simulink model "model"  (R2017b)
settings: Solver=ode23tb  StartTime=0.0  StopTime=0.3  EnableMultiTasking=on
InitFcn:
  | initializer_assignment4
values from neighbouring files (symbols this model uses):
  C = 15e-06    (= 1.5e-05)    [main.m]
  Iqref = 0    [main.m]
  K_cross = (L_inv) * 2*pi*f_sin    (= 0.785398163397)    [main.m]
  Kc = 1/(w_z/K * Gc)    [main.m]
  Ki = 2776    [main.m]
  Kp = 1.165    [main.m]
  L_a_grid = L_grid    (= 0.0015)    [main.m]
  L_a_inv = L_inv    (= 0.0025)    [main.m]
  L_b_grid = L_grid    (= 0.0015)    [main.m]
  L_b_inv = L_inv    (= 0.0025)    [main.m]
  L_c_grid = L_grid    (= 0.0015)    [main.m]
  L_c_inv = L_inv    (= 0.0025)    [main.m]
  m_a = 1/Gpwm    (= 0.00285714285714)    [main.m]
  R_d = 3.1    [main.m]
  V_ac = 400    [main.m]
  w_p = w_cr * K    [main.m]
  w_ref = f_sin*2*pi    (= 314.159265359)    [main.m]
  w_z = w_cr / K    [main.m]
libraries: powerlib x20, powerlib_meascontrol x5
settings Model: Creator=Daniele  LastModifiedBy=izzy
settings SolverCC: ZeroCrossAlgorithm=Adaptive
settings DataIOCC: LimitDataPoints=on  SaveFormat=Array
settings OptimizationCC: LifeSpan=inf
settings DebuggingCC: UnderspecifiedInitializationDetection=Classic  MergeDetectMultiDrivingBlocksExec=none  SolverPrmCheckMsg=warning  SFUnexpectedBacktrackingDiag=warning  SFNoUnconditionalDefaultTransitionDiag=warning  SFExecutionAtInitializationDiag=none
settings HardwareCC: ProdBitPerPointer=32  ProdBitPerSizeT=32  ProdBitPerPtrDiffT=32  ProdLargestAtomicFloat=None  ProdIntDivRoundTo=Undefined  ProdEndianess=Unspecified  ProdWordSize=32  ProdHWDeviceType=32-bit Generic
settings ModelReferenceCC: PropagateSignalLabelsOutOfModel=off
settings CodeAppCC: StateflowObjectComments=on
settings GRTTargetCC: TargetLangStandard=C89/C90 (ANSI)  GeneratePreprocessorConditionals=Disable all
settings ConfigComp: CovMetricSettings=dw  CovHtmlReporting=on  CovSaveCumulativeToWorkspaceVar=on  CovSaveSingleToWorkspaceVar=on  CovExternalEMLEnable=off
settings SimscapeCC: SimscapeNormalizeSystem=off

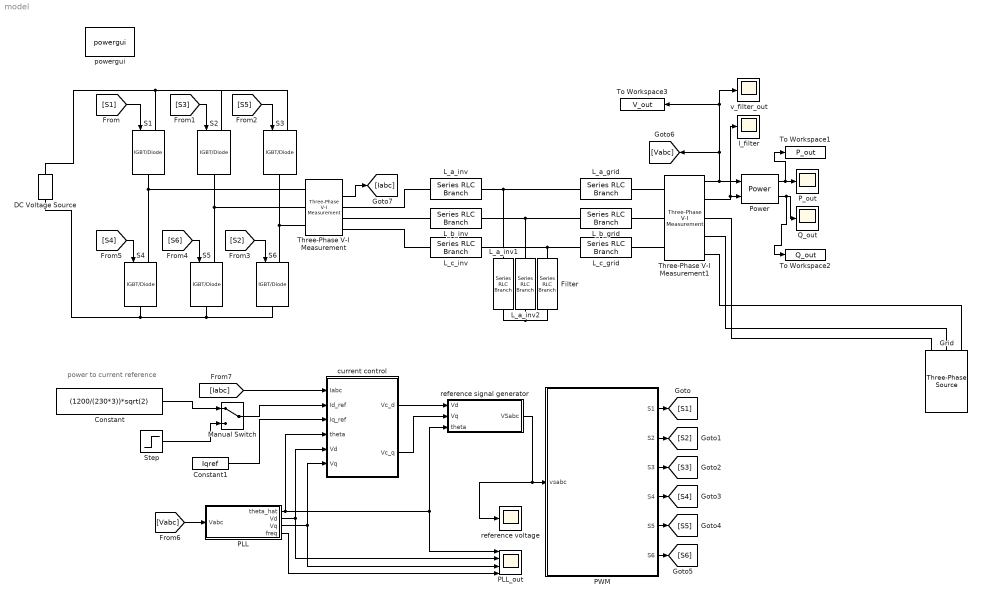
== system model ==
  note: power to current reference
  Constant : Constant  Value=(1200/(230*3))*sqrt(2)
  Constant1 : Constant  Value=Iqref
  DC Voltage Source : powerlib/Electrical Sources/DC Voltage Source  Amplitude=700  Measurements=None
  Filter : powerlib/Elements/Series RLC Branch  LConnTagsString=__new0  RConnTagsString=__new0  BranchType=RC  Resistance=R_d  Inductance=L_a_inv  SetiL0=off  InitialCurrent=0  Capacitance=C  Setx0=off  InitialVoltage=0  Measurements=None
  Grid : powerlib/Electrical Sources/Three-Phase Source  InternalConnection=Yg  VoltagePhases=off  Voltage=V_ac  PhaseAngle=0  Voltage_phases=[25e3 25e3 25e3]/sqrt(3)  PhaseAngles_phases=[0 -120 +120]  Frequency=50  NonIdealSource=on  SpecifyImpedance=off  Resistance=0.48  Inductance=250e-6  ShortCircuitLevel=100e6  BaseVoltage=V_ac  XRratio=7  BusType=swing  Pref=0  Qref=0  Prefabc=[10e3, 10e3, 10e3]  Qrefabc=[0, 0, 0]  Qmin=-inf  Qmax=inf
  I_filter : Scope
  L_a_grid : powerlib/Elements/Series RLC Branch  LConnTagsString=__new0  RConnTagsString=__new0  BranchType=L  Resistance=1  Inductance=L_a_grid  SetiL0=off  InitialCurrent=0  Capacitance=0  Setx0=off  InitialVoltage=0  Measurements=None
  L_a_inv : powerlib/Elements/Series RLC Branch  LConnTagsString=__new0  RConnTagsString=__new0  BranchType=L  Resistance=1  Inductance=L_a_inv  SetiL0=off  InitialCurrent=0  Capacitance=0  Setx0=off  InitialVoltage=0  Measurements=None
  L_a_inv1 : powerlib/Elements/Series RLC Branch  LConnTagsString=__new0  RConnTagsString=__new0  BranchType=RC  Resistance=R_d  Inductance=L_a_inv  SetiL0=off  InitialCurrent=0  Capacitance=C  Setx0=off  InitialVoltage=0  Measurements=None
  L_a_inv2 : powerlib/Elements/Series RLC Branch  LConnTagsString=__new0  RConnTagsString=__new0  BranchType=RC  Resistance=R_d  Inductance=L_a_inv  SetiL0=off  InitialCurrent=0  Capacitance=C  Setx0=off  InitialVoltage=0  Measurements=None
  L_b_grid : powerlib/Elements/Series RLC Branch  LConnTagsString=__new0  RConnTagsString=__new0  BranchType=L  Resistance=1  Inductance=L_b_grid  SetiL0=off  InitialCurrent=0  Capacitance=0  Setx0=off  InitialVoltage=0  Measurements=None
  L_b_inv : powerlib/Elements/Series RLC Branch  LConnTagsString=__new0  RConnTagsString=__new0  BranchType=L  Resistance=1  Inductance=L_b_inv  SetiL0=off  InitialCurrent=0  Capacitance=0  Setx0=off  InitialVoltage=0  Measurements=None
  L_c_grid : powerlib/Elements/Series RLC Branch  LConnTagsString=__new0  RConnTagsString=__new0  BranchType=L  Resistance=1  Inductance=L_c_grid  SetiL0=off  InitialCurrent=0  Capacitance=0  Setx0=off  InitialVoltage=0  Measurements=None
  L_c_inv : powerlib/Elements/Series RLC Branch  LConnTagsString=__new0  RConnTagsString=__new0  BranchType=L  Resistance=1  Inductance=L_c_inv  SetiL0=off  InitialCurrent=0  Capacitance=0  Setx0=off  InitialVoltage=0  Measurements=None
  Manual Switch : ManualSwitch
  PLL : Subsystem
  PLL_out : Scope  NumInputPorts=4
  PWM : Subsystem
  P_out : Scope
  Power : powerlib_meascontrol/Measurements/Power  Freq=f_sin  Vinit=[1, 0]  Iinit=[1, 0]  Ts=0
      settings: SourceProductName=Simscape Power Systems
  Q_out : Scope
  S{1..6} (6 alike) : powerlib/Power Electronics/IGBT//Diode  Ron=1e-3  Rs=1e5  Cs=inf  Measurements=off
  Step : Step  Time=0.15  Before=40  After=0  SampleTime=0
  Three-Phase V-I Measurement : powerlib/Measurements/Three-Phase V-I Measurement  VoltageMeasurement=phase-to-ground  SetLabelV=off  LabelV=Vabc  Vpu=off  VpuLL=off  CurrentMeasurement=yes  SetLabelI=off  LabelI=Iabc  Ipu=off  Pbase=100e6  Vbase=500e3  OutputType=Complex  PhasorSimulation=off  PSBequivalent=0
  Three-Phase V-I Measurement1 : powerlib/Measurements/Three-Phase V-I Measurement  VoltageMeasurement=phase-to-ground  SetLabelV=off  LabelV=Vabc  Vpu=off  VpuLL=off  CurrentMeasurement=yes  SetLabelI=off  LabelI=Iabc  Ipu=off  Pbase=100e6  Vbase=500e3  OutputType=Complex  PhasorSimulation=off  PSBequivalent=0
  To Workspace1 : ToWorkspace  VariableName=P_out  SaveFormat=Timeseries  SampleTime=-1
  To Workspace2 : ToWorkspace  VariableName=Q_out  SaveFormat=Timeseries  SampleTime=-1
  To Workspace3 : ToWorkspace  VariableName=V_out  SaveFormat=Timeseries  SampleTime=-1
  current control : Subsystem
  powergui : powerlib/powergui  Priority=1  SimulationMode=Discrete  SampleTime=0.000001  frequency=50  Iterations=50  frequencyindice=50  Pbase=100e6  ErrMax=1e-4  UnitsV=kV  UnitsW=MW  buscounter=0  FunctionMessages=off  echomessages=off  EnableUseOfTLC=off  CurrentSourceSwitches=off  DisableSnubberDevices=off  DisableRonSwitches=off  DisableVfSwitches=off  DisplayEquations=off  SolverType=Tustin/Backward Euler (TBE)  Interpol=off  ExternalGateDelay=off  methode=off  Ts=0  x0status=blocks  SPID=off  SwTol=0  HookPort=off  RestoreLinks=warning  ResistiveCurrentMeasurement=off  Frange=[0:2:500]  Ylog=off  Xlog=on  ShowGrid=off  save=off  variable=ZData  structure=0  ZoomFFT=off  StartTime=0.0  cycles=1  DisplayStyle=1  fundamental=60  FreqAxis=off  MaxFrequency=1000  frequencyindicesteady=1  RmsSteady=1  display=off
  reference signal generator : Subsystem
  reference voltage : Scope
  v_filter_out : Scope
  wires:
  Three-Phase V-I Measurement/2 -> [Iabc]
  [S1] -> S1/1
  [S3] -> S2/1
  [S5] -> S3/1
  [S2] -> S6/1
  [S6] -> S5/1
  [S4] -> S4/1
  reference signal generator/1(VSabc) -> reference voltage/1, PWM/1(vsabc)
  PWM/1(S1) -> [S1]
  PWM/2(S2) -> [S2]
  PWM/3(S3) -> [S3]
  PWM/4(S4) -> [S4]
  PWM/5(S5) -> [S5]
  PWM/6(S6) -> [S6]
  Three-Phase V-I Measurement1/2 -> I_filter/1, Power/2
  Three-Phase V-I Measurement1/1 -> To Workspace3/1, v_filter_out/1, [Vabc], Power/1
  [Vabc] -> PLL/1(Vabc)
  PLL/1(theta_hat) -> reference signal generator/3(theta), PLL_out/1, current control/4(theta)
  PLL/2(Vd) -> PLL_out/2, current control/5(Vd)
  PLL/3(Vq) -> PLL_out/3, current control/6(Vq)
  PLL/4(freq) -> PLL_out/4
  current control/1(Vc_d) -> reference signal generator/1(Vd)
  current control/2(Vc_q) -> reference signal generator/2(Vq)
  [Iabc] -> current control/1(Iabc)
  Constant1/1 -> current control/3(Iq_ref)
  Manual Switch/1 -> current control/2(Id_ref)
  Step/1 -> Manual Switch/2
  Constant/1 -> Manual Switch/1
  Power/1 -> To Workspace1/1, P_out/1
  Power/2 -> To Workspace2/1, Q_out/1
  connections:
  L_a_inv/LConn1 -- L_a_inv1/LConn1 -- L_a_grid/RConn1
  L_b_inv/LConn1 -- L_a_inv2/LConn1 -- L_b_grid/RConn1
  L_c_inv/LConn1 -- Filter/LConn1 -- L_c_grid/RConn1
  L_a_inv1/RConn1 -- L_a_inv2/RConn1 -- Filter/RConn1
  S1/RConn1 -- S4/LConn1 -- Three-Phase V-I Measurement/LConn1
  S2/RConn1 -- S5/LConn1 -- Three-Phase V-I Measurement/LConn2
  S3/RConn1 -- S6/LConn1 -- Three-Phase V-I Measurement/LConn3
  S3/LConn1 -- S2/LConn1 -- DC Voltage Source/RConn1 -- S1/LConn1
  S4/RConn1 -- DC Voltage Source/LConn1 -- S6/RConn1 -- S5/RConn1
  Three-Phase V-I Measurement/RConn1 -- L_a_inv/RConn1
  Three-Phase V-I Measurement/RConn2 -- L_b_inv/RConn1
  Three-Phase V-I Measurement/RConn3 -- L_c_inv/RConn1
  Three-Phase V-I Measurement1/LConn1 -- L_a_grid/LConn1
  L_b_grid/LConn1 -- Three-Phase V-I Measurement1/LConn2
  L_c_grid/LConn1 -- Three-Phase V-I Measurement1/LConn3
  Grid/RConn1 -- Three-Phase V-I Measurement1/RConn1
  Grid/RConn2 -- Three-Phase V-I Measurement1/RConn2
  Grid/RConn3 -- Three-Phase V-I Measurement1/RConn3

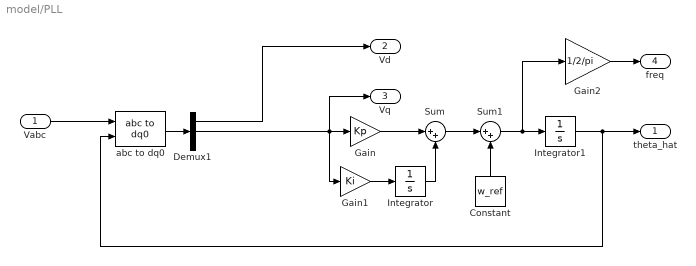
== system model/PLL ==
  Vabc : Inport
  Constant : Constant  Value=w_ref
  Demux1 : Demux  Outputs=3
  Gain : Gain  Gain=Kp
  Gain1 : Gain  Gain=Ki
  Gain2 : Gain  Gain=1/2/pi
  Integrator : Integrator
  Integrator1 : Integrator
  Sum : Sum  Inputs=|++
  Sum1 : Sum  Inputs=|++
  abc to dq0 : powerlib_meascontrol/Transformations/abc to dq0  Alignment=90 degrees behind phase A axis
  theta_hat : Outport
  Vd : Outport  Port=2
  Vq : Outport  Port=3
  freq : Outport  Port=4
  wires:
  Gain1/1 -> Integrator/1
  Gain/1 -> Sum/1
  Integrator/1 -> Sum/2
  Constant/1 -> Sum1/2
  Sum/1 -> Sum1/1
  Sum1/1 -> Gain2/1, Integrator1/1
  Integrator1/1 -> abc to dq0/2, theta_hat/1
  Vabc/1 -> abc to dq0/1
  Gain2/1 -> freq/1
  Demux1/2 -> Vq/1, Gain1/1, Gain/1
  Demux1/1 -> Vd/1
  abc to dq0/1 -> Demux1/1

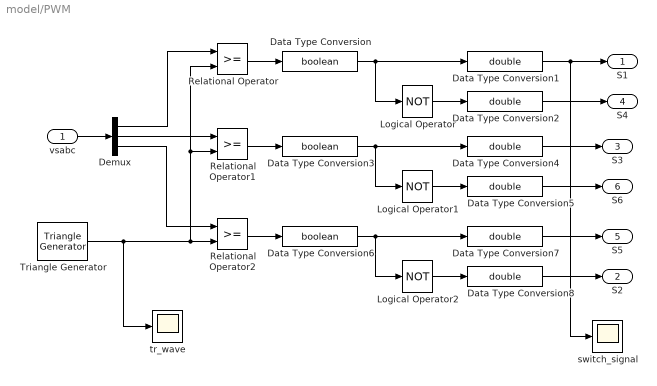
== system model/PWM ==
  vsabc : Inport
  Data Type Conversion : DataTypeConversion  OutDataTypeStr=boolean
  Data Type Conversion{1..2,4..5,7..8} (6 alike) : DataTypeConversion  OutDataTypeStr=double
  Data Type Conversion3 : DataTypeConversion  OutDataTypeStr=boolean
  Data Type Conversion6 : DataTypeConversion  OutDataTypeStr=boolean
  Demux : Demux  Outputs=3
  Logical Operator : Logic  Operator=NOT  AllPortsSameDT=off  OutDataTypeStr=boolean
  Logical Operator1 : Logic  Operator=NOT  AllPortsSameDT=off  OutDataTypeStr=boolean
  Logical Operator2 : Logic  Operator=NOT  AllPortsSameDT=off  OutDataTypeStr=boolean
  Relational Operator : RelationalOperator  OutDataTypeStr=boolean  RndMeth=Nearest
  Relational Operator1 : RelationalOperator  OutDataTypeStr=boolean  RndMeth=Nearest
  Relational Operator2 : RelationalOperator  OutDataTypeStr=boolean  RndMeth=Nearest
  Triangle Generator : powerlib_meascontrol/Pulse & Signal Generators/Triangle Generator  Freq=f_carrier  Phase=0  Ts=0
  switch_signal : Scope
  tr_wave : Scope
  S1 : Outport
  S2 : Outport  Port=2
  S3 : Outport  Port=3
  S4 : Outport  Port=4
  S5 : Outport  Port=5
  S6 : Outport  Port=6
  wires:
  vsabc/1 -> Demux/1
  Relational Operator/1 -> Data Type Conversion/1
  Demux/1 -> Relational Operator/1
  Data Type Conversion1/1 -> switch_signal/1, S1/1
  Data Type Conversion2/1 -> S4/1
  Data Type Conversion/1 -> Logical Operator/1, Data Type Conversion1/1
  Logical Operator/1 -> Data Type Conversion2/1
  Relational Operator1/1 -> Data Type Conversion3/1
  Demux/2 -> Relational Operator1/1
  Data Type Conversion4/1 -> S3/1
  Data Type Conversion3/1 -> Logical Operator1/1, Data Type Conversion4/1
  Logical Operator1/1 -> Data Type Conversion5/1
  Relational Operator2/1 -> Data Type Conversion6/1
  Demux/3 -> Relational Operator2/1
  Data Type Conversion7/1 -> S5/1
  Data Type Conversion8/1 -> S2/1
  Data Type Conversion6/1 -> Logical Operator2/1, Data Type Conversion7/1
  Logical Operator2/1 -> Data Type Conversion8/1
  Triangle Generator/1 -> tr_wave/1, Relational Operator/2, Relational Operator1/2, Relational Operator2/2
  Data Type Conversion5/1 -> S6/1

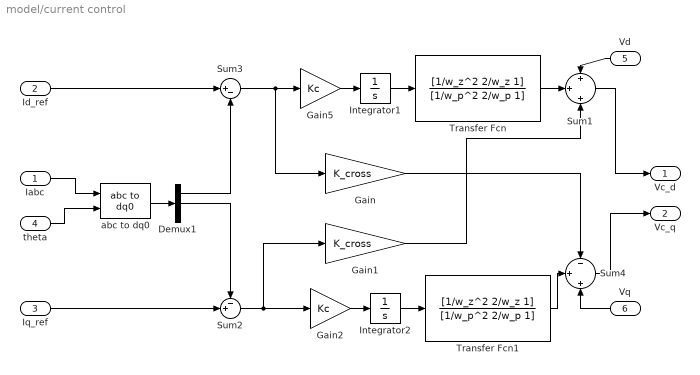
== system model/current control ==
  Iabc : Inport
  Id_ref : Inport  Port=2
  Iq_ref : Inport  Port=3
  theta : Inport  Port=4
  Vd : Inport  Port=5
  Vq : Inport  Port=6
  Demux1 : Demux  Outputs=3
  Gain : Gain  Gain=K_cross
  Gain1 : Gain  Gain=K_cross
  Gain2 : Gain  Gain=Kc
  Gain5 : Gain  Gain=Kc
  Integrator1 : Integrator
  Integrator2 : Integrator
  Sum1 : Sum  Inputs=+|+|+
  Sum2 : Sum  Inputs=-+|
  Sum3 : Sum  Inputs=|+-
  Sum4 : Sum  Inputs=-|+|+
  Transfer Fcn : TransferFcn  Numerator=[1/w_z^2 2/w_z 1]  Denominator=[1/w_p^2 2/w_p 1]
  Transfer Fcn1 : TransferFcn  Numerator=[1/w_z^2 2/w_z 1]  Denominator=[1/w_p^2 2/w_p 1]
  abc to dq0 : powerlib_meascontrol/Transformations/abc to dq0  Alignment=90 degrees behind phase A axis
  Vc_d : Outport
  Vc_q : Outport  Port=2
  wires:
  Sum1/1 -> Vc_d/1
  abc to dq0/1 -> Demux1/1
  theta/1 -> abc to dq0/2
  Vd/1 -> Sum1/1
  Demux1/2 -> Sum2/1
  Iq_ref/1 -> Sum2/2
  Demux1/1 -> Sum3/2
  Id_ref/1 -> Sum3/1
  Iabc/1 -> abc to dq0/1
  Vq/1 -> Sum4/3
  Gain/1 -> Sum4/1
  Gain1/1 -> Sum1/3
  Sum3/1 -> Gain/1, Gain5/1
  Gain5/1 -> Integrator1/1
  Transfer Fcn/1 -> Sum1/2
  Integrator1/1 -> Transfer Fcn/1
  Sum4/1 -> Vc_q/1
  Sum2/1 -> Gain2/1, Gain1/1
  Gain2/1 -> Integrator2/1
  Integrator2/1 -> Transfer Fcn1/1
  Transfer Fcn1/1 -> Sum4/2

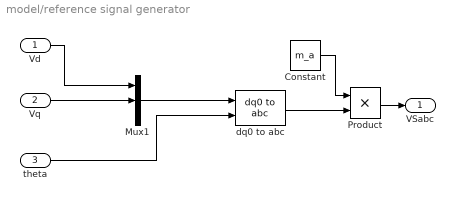
== system model/reference signal generator ==
  Vd : Inport
  Vq : Inport  Port=2
  theta : Inport  Port=3
  Constant : Constant  Value=m_a
  Mux1 : Mux  Inputs=3
  Product : Product
  dq0 to abc : powerlib_meascontrol/Transformations/dq0 to abc  Alignment=90 degrees behind phase A axis
  VSabc : Outport
  wires:
  Vd/1 -> Mux1/1
  Vq/1 -> Mux1/2
  Constant/1 -> Product/1
  Product/1 -> VSabc/1
  Mux1/1 -> dq0 to abc/1
  theta/1 -> dq0 to abc/2
  dq0 to abc/1 -> Product/2
